simulink model "crazyflie"  (R2018b)
settings: Solver=VariableStepAuto  StartTime=0.0  StopTime=40  FixedStep=Ts  RelTol=1e-10
values from neighbouring files (symbols this model uses):
  bf = 1.28192e-08    [matlab.mat]    (also in model_init.m; work.mat)
  bm = 8.06428e-05    [matlab.mat]    (also in model_init.m; work.mat)
  c_10 = 0.5    [matlab.mat]    (also in model_init.m; work.mat)
  c_11 = 2    [matlab.mat]    (also in model_init.m; work.mat)
  c_12 = 0.5    [matlab.mat]    (also in model_init.m; work.mat)
  c_9 = 2    [matlab.mat]    (also in model_init.m; work.mat)
  g = 9.81    [matlab.mat]    (also in model_init.m; work.mat)
  Ix = 1.657171e-05    [matlab.mat]    (also in model_init.m; work.mat)
  Iy = 1.657171e-05    [matlab.mat]    (also in model_init.m; work.mat)
  Iz = 2.9261652e-05    [matlab.mat]    (also in model_init.m; work.mat)
  kdp = 0.03    [matlab.mat]    (also in model_init.m = 0.1; work.mat = 0.1)
  kdps = 0.01    [matlab.mat]    (also in model_init.m = 0.001; work.mat = 0.001)
  kdt = 0.03    [matlab.mat]    (also in model_init.m = 0.1; work.mat = 0.1)
  kdz = 3    [matlab.mat]    (also in model_init.m = 8; work.mat = 8)
  kiz = 2    [matlab.mat]    (also in model_init.m = 3; work.mat = 3)
  kpp = 0.03    [matlab.mat]    (also in model_init.m = 0.2; work.mat = 0.2)
  kpps = 0.01    [matlab.mat]    (also in model_init.m = 0.001; work.mat = 0.001)
  kpt = 0.03    [matlab.mat]    (also in model_init.m = 1; work.mat = 1)
  kpz = 2    [matlab.mat]    (also in model_init.m = 15; work.mat = 15)
  l = 0.046    [matlab.mat]    (also in model_init.m; work.mat)
  lambda_5 = 0.015    [matlab.mat]    (also in model_init.m; work.mat)
  lambda_6 = 0.015    [matlab.mat]    (also in model_init.m; work.mat)
  m = 0.027    [matlab.mat]    (also in model_init.m; work.mat)
  phi_ic = phi(end)    [Crazyflie_simulation.m]    (also in work.mat = 1.92698500832e-08)
  psi_ic = psi(end)    [Crazyflie_simulation.m]    (also in work.mat = 2.27785803884e-19)
  psi_r = 0    [Crazyflie_simulation.m]    (also in work.mat)
  sigma1_ic = sigma_1(end)    [Crazyflie_simulation.m]    (also in work.mat = 2272.7745434)
  sigma2_ic = sigma_2(end)    [Crazyflie_simulation.m]    (also in work.mat = 2272.7745434)
  sigma3_ic = sigma_3(end)    [Crazyflie_simulation.m]    (also in work.mat = 2272.77454331)
  sigma4_ic = sigma_4(end)    [Crazyflie_simulation.m]    (also in work.mat = 2272.77454331)
  Sigma_max = 2618    [matlab.mat]    (also in model_init.m; work.mat)
  T_m = 0.0125    [matlab.mat]    (also in model_init.m; work.mat)
  theta_ic = theta(end)    [Crazyflie_simulation.m]    (also in work.mat = 4.295907714e-08)
  x_ic = x(end)    [Crazyflie_simulation.m]    (also in work.mat = -0.000112604495344)
  x_r = 10*rrt_trajectory(i,1)/map_dimension(1)    [Crazyflie_simulation.m]    (also in matlab.mat = 1; work.mat = 0)
  y_ic = y(end)    [Crazyflie_simulation.m]    (also in work.mat = 9.00005076367)
  y_r = 10*rrt_trajectory(i,2)/map_dimension(2)    [Crazyflie_simulation.m]    (also in matlab.mat = 1; work.mat = 9)
  z_ic = z(end)    [Crazyflie_simulation.m]    (also in work.mat = 0.999916821767)
  z_r = 1    [Crazyflie_simulation.m]    (also in work.mat)
settings Model: Creator=alessandrosebastianelli  LastModifiedBy=alessandrosebastianelli
settings SFSimCC: SimUseLocalCustomCode=off
settings RTWCC: RTWUseLocalCustomCode=off

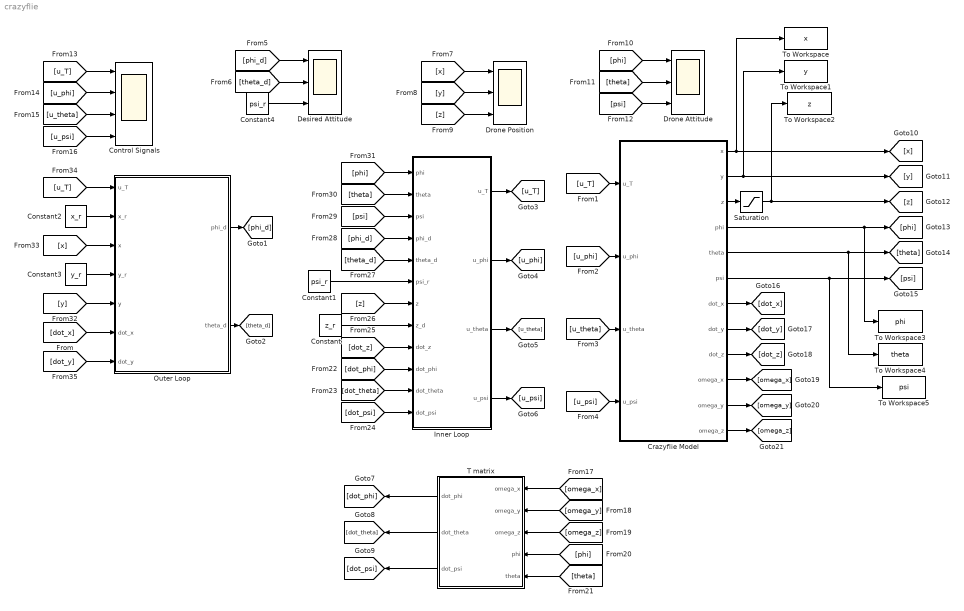
== system crazyflie ==
  Constant : Constant  Value=z_r
  Constant1 : Constant  Value=psi_r
  Constant2 : Constant  Value=x_r
  Constant3 : Constant  Value=y_r
  Constant4 : Constant  Value=psi_r
  Control Signals : Scope  NumInputPorts=4
  Crazyflie Model : Subsystem
  Desired Attitude : Scope  NumInputPorts=3
  Drone Attitude : Scope  NumInputPorts=3
  Drone Position : Scope  NumInputPorts=3
  Inner Loop : Subsystem
  Outer Loop : Subsystem
  Saturation : Saturate  UpperLimit=inf  LowerLimit=0
  T matrix : Subsystem
  To Workspace : ToWorkspace  VariableName=x  SampleTime=-1
  To Workspace1 : ToWorkspace  VariableName=y  SampleTime=-1
  To Workspace2 : ToWorkspace  VariableName=z  SampleTime=-1
  To Workspace3 : ToWorkspace  VariableName=phi  SampleTime=-1
  To Workspace4 : ToWorkspace  VariableName=theta  SampleTime=-1
  To Workspace5 : ToWorkspace  VariableName=psi  SampleTime=-1
  wires:
  Constant1/1 -> Inner Loop/6(psi_r)
  [dot_x] -> Outer Loop/6(dot_x)
  Outer Loop/2(theta_d) -> [theta_d]
  T matrix/1(dot_phi) -> [dot_phi]
  T matrix/2(dot_theta) -> [dot_theta]
  T matrix/3(dot_psi) -> [dot_psi]
  Inner Loop/1(u_T) -> [u_T]
  Inner Loop/2(u_phi) -> [u_phi]
  Inner Loop/3(u_theta) -> [u_theta]
  Inner Loop/4(u_psi) -> [u_psi]
  [u_T] -> Crazyflie Model/1(u_T)
  [u_phi] -> Crazyflie Model/2(u_phi)
  [u_theta] -> Crazyflie Model/3(u_theta)
  [u_psi] -> Crazyflie Model/4(u_psi)
  Crazyflie Model/1(x) -> [x], To Workspace/1
  Crazyflie Model/2(y) -> To Workspace1/1, [y]
  Crazyflie Model/3(z) -> Saturation/1
  Crazyflie Model/4(phi) -> To Workspace3/1, [phi]
  Crazyflie Model/5(theta) -> To Workspace4/1, [theta]
  Crazyflie Model/6(psi) -> To Workspace5/1, [psi]
  Crazyflie Model/7(dot_x) -> [dot_x]
  Crazyflie Model/8(dot_y) -> [dot_y]
  Crazyflie Model/9(dot_z) -> [dot_z]
  Crazyflie Model/10(omega_x) -> [omega_x]
  Crazyflie Model/11(omega_y) -> [omega_y]
  Crazyflie Model/12(omega_z) -> [omega_z]
  [phi_d] -> Desired Attitude/1
  [theta_d] -> Desired Attitude/2
  Constant4/1 -> Desired Attitude/3
  [z] -> Drone Position/3
  [y] -> Drone Position/2
  [x] -> Drone Position/1
  [phi] -> Drone Attitude/1
  [theta] -> Drone Attitude/2
  [psi] -> Drone Attitude/3
  [u_T] -> Control Signals/1
  [u_phi] -> Control Signals/2
  [u_theta] -> Control Signals/3
  [u_psi] -> Control Signals/4
  [omega_y] -> T matrix/2(omega_y)
  [omega_x] -> T matrix/1(omega_x)
  [omega_z] -> T matrix/3(omega_z)
  [phi] -> T matrix/4(phi)
  [theta] -> T matrix/5(theta)
  [dot_phi] -> Inner Loop/10(dot_phi)
  [dot_psi] -> Inner Loop/12(dot_psi)
  [dot_theta] -> Inner Loop/11(dot_theta)
  [dot_z] -> Inner Loop/9(dot_z)
  [z] -> Inner Loop/7(z)
  [phi] -> Inner Loop/1(phi)
  [theta] -> Inner Loop/2(theta)
  [psi] -> Inner Loop/3(psi)
  [phi_d] -> Inner Loop/4(phi_d)
  [theta_d] -> Inner Loop/5(theta_d)
  [u_T] -> Outer Loop/1("u_T ")
  [x] -> Outer Loop/3(x)
  [y] -> Outer Loop/5(y)
  Outer Loop/1(phi_d) -> [phi_d]
  [dot_y] -> Outer Loop/7(dot_y)
  Saturation/1 -> To Workspace2/1, [z]
  Constant2/1 -> Outer Loop/2(x_r)
  Constant3/1 -> Outer Loop/4(y_r)
  Constant/1 -> Inner Loop/8(z_d)

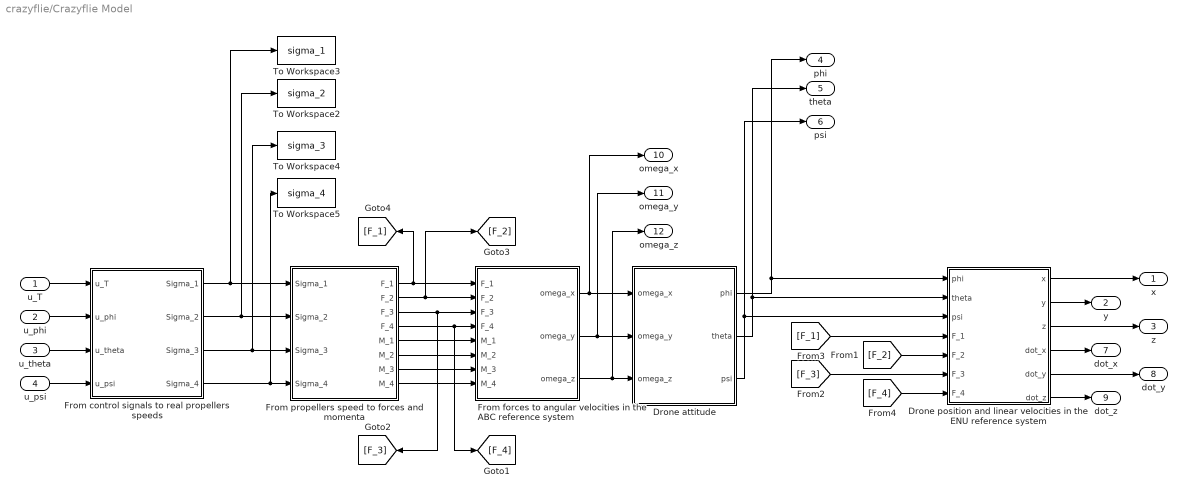
== system crazyflie/Crazyflie Model ==
  u_T : Inport
  u_phi : Inport  Port=2
  u_theta : Inport  Port=3
  u_psi : Inport  Port=4
  Drone attitude : Subsystem
  Drone position and linear velocities in the ENU reference system : Subsystem
  From control signals to real propellers speeds : Subsystem
  From forces to angular velocities in the ABC reference system : Subsystem
  From propellers speed to forces and momenta : Subsystem
  To Workspace2 : ToWorkspace  VariableName=sigma_2  SampleTime=-1
  To Workspace3 : ToWorkspace  VariableName=sigma_1  SampleTime=-1
  To Workspace4 : ToWorkspace  VariableName=sigma_3  SampleTime=-1
  To Workspace5 : ToWorkspace  VariableName=sigma_4  SampleTime=-1
  x : Outport
  y : Outport  Port=2
  z : Outport  Port=3
  phi : Outport  Port=4
  theta : Outport  Port=5
  psi : Outport  Port=6
  dot_x : Outport  Port=7
  dot_y : Outport  Port=8
  dot_z : Outport  Port=9
  omega_x : Outport  Port=10
  omega_y : Outport  Port=11
  omega_z : Outport  Port=12
  wires:
  u_T/1 -> From control signals to real propellers speeds/1(u_T)
  u_phi/1 -> From control signals to real propellers speeds/2(u_phi)
  u_theta/1 -> From control signals to real propellers speeds/3(u_theta)
  u_psi/1 -> From control signals to real propellers speeds/4(u_psi)
  From control signals to real propellers speeds/1(Sigma_1) -> To Workspace3/1, From propellers speed to forces and momenta/1(Sigma_1)
  From control signals to real propellers speeds/2(Sigma_2) -> To Workspace2/1, From propellers speed to forces and momenta/2(Sigma_2)
  From control signals to real propellers speeds/3(Sigma_3) -> To Workspace4/1, From propellers speed to forces and momenta/3(Sigma_3)
  From control signals to real propellers speeds/4(Sigma_4) -> To Workspace5/1, From propellers speed to forces and momenta/4(Sigma_4)
  From propellers speed to forces and momenta/1(F_1) -> [F_1], From forces to angular velocities in the ABC reference system/1(F_1)
  From propellers speed to forces and momenta/2(F_2) -> [F_2], From forces to angular velocities in the ABC reference system/2(F_2)
  From propellers speed to forces and momenta/3(F_3) -> [F_3], From forces to angular velocities in the ABC reference system/3(F_3)
  From propellers speed to forces and momenta/4(F_4) -> [F_4], From forces to angular velocities in the ABC reference system/4(F_4)
  From propellers speed to forces and momenta/5(M_1) -> From forces to angular velocities in the ABC reference system/5(M_1)
  From propellers speed to forces and momenta/6(M_2) -> From forces to angular velocities in the ABC reference system/6(M_2)
  From propellers speed to forces and momenta/7(M_3) -> From forces to angular velocities in the ABC reference system/7(M_3)
  From propellers speed to forces and momenta/8(M_4) -> From forces to angular velocities in the ABC reference system/8(M_4)
  From forces to angular velocities in the ABC reference system/1(omega_x) -> omega_x/1, Drone attitude/1(omega_x)
  From forces to angular velocities in the ABC reference system/2(omega_y) -> omega_y/1, Drone attitude/2(omega_y)
  From forces to angular velocities in the ABC reference system/3(omega_z) -> omega_z/1, Drone attitude/3(omega_z)
  Drone position and linear velocities in the ENU reference system/1(x) -> x/1
  Drone position and linear velocities in the ENU reference system/2(y) -> y/1
  Drone position and linear velocities in the ENU reference system/3(z) -> z/1
  Drone position and linear velocities in the ENU reference system/4(dot_x) -> dot_x/1
  Drone position and linear velocities in the ENU reference system/5(dot_y) -> dot_y/1
  Drone position and linear velocities in the ENU reference system/6(dot_z) -> dot_z/1
  Drone attitude/1(phi) -> Drone position and linear velocities in the ENU reference system/1(phi), phi/1
  Drone attitude/2(theta) -> Drone position and linear velocities in the ENU reference system/2(theta), theta/1
  Drone attitude/3(psi) -> Drone position and linear velocities in the ENU reference system/3(psi), psi/1
  [F_1] -> Drone position and linear velocities in the ENU reference system/4(F_1)
  [F_2] -> Drone position and linear velocities in the ENU reference system/5(F_2)
  [F_3] -> Drone position and linear velocities in the ENU reference system/6(F_3)
  [F_4] -> Drone position and linear velocities in the ENU reference system/7(F_4)

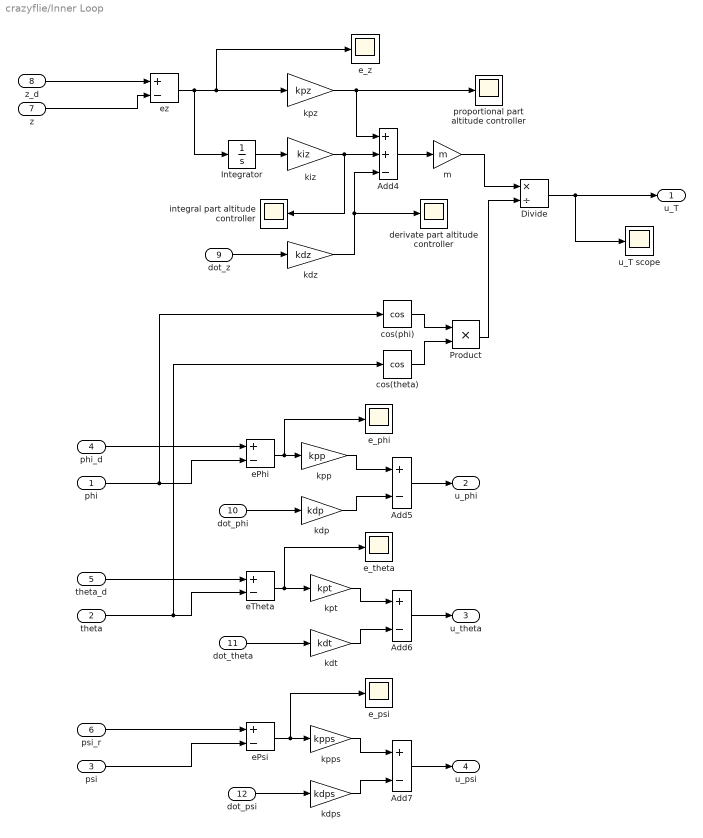
== system crazyflie/Inner Loop ==
  phi : Inport
  theta : Inport  Port=2
  psi : Inport  Port=3
  phi_d : Inport  Port=4
  theta_d : Inport  Port=5
  psi_r : Inport  Port=6
  z : Inport  Port=7
  z_d : Inport  Port=8
  dot_z : Inport  Port=9
  dot_phi : Inport  Port=10
  dot_theta : Inport  Port=11
  dot_psi : Inport  Port=12
  Add4 : Sum  Inputs=++-
  Add5 : Sum  Inputs=+-
  Add6 : Sum  Inputs=+-
  Add7 : Sum  Inputs=+-
  Divide : Product  Inputs=*/
  Integrator : Integrator
  Product : Product  RndMeth=Zero
  cos(phi) : Trigonometry  Operator=cos
  cos(theta) : Trigonometry  Operator=cos
  derivate part altitude controller : Scope
  ePhi : Sum  Inputs=+-
  ePsi : Sum  Inputs=+-
  eTheta : Sum  Inputs=+-
  e_phi : Scope
  e_psi : Scope
  e_theta : Scope
  e_z : Scope
  ez : Sum  Inputs=+-
  integral part altitude controller : Scope
  kdp : Gain  Gain=kdp
  kdps : Gain  Gain=kdps
  kdt : Gain  Gain=kdt
  kdz : Gain  Gain=kdz
  kiz : Gain  Gain=kiz
  kpp : Gain  Gain=kpp
  kpps : Gain  Gain=kpps
  kpt : Gain  Gain=kpt
  kpz : Gain  Gain=kpz
  m : Gain  Gain=m
  proportional part altitude controller : Scope
  u_T scope : Scope
  u_T : Outport
  u_phi : Outport  Port=2
  u_theta : Outport  Port=3
  u_psi : Outport  Port=4
  wires:
  phi/1 -> ePhi/2, cos(phi)/1
  theta/1 -> eTheta/2, cos(theta)/1
  psi/1 -> ePsi/2
  phi_d/1 -> ePhi/1
  theta_d/1 -> eTheta/1
  psi_r/1 -> ePsi/1
  ePhi/1 -> e_phi/1, kpp/1
  dot_phi/1 -> kdp/1
  eTheta/1 -> e_theta/1, kpt/1
  dot_theta/1 -> kdt/1
  ePsi/1 -> e_psi/1, kpps/1
  dot_psi/1 -> kdps/1
  z/1 -> ez/2
  z_d/1 -> ez/1
  ez/1 -> Integrator/1, kpz/1, e_z/1
  dot_z/1 -> kdz/1
  kpz/1 -> proportional part altitude controller/1, Add4/1
  kdz/1 -> Add4/3, derivate part altitude controller/1
  kpp/1 -> Add5/1
  kdp/1 -> Add5/2
  Add5/1 -> u_phi/1
  kpt/1 -> Add6/1
  kdt/1 -> Add6/2
  Add6/1 -> u_theta/1
  kpps/1 -> Add7/1
  kdps/1 -> Add7/2
  Add7/1 -> u_psi/1
  cos(phi)/1 -> Product/1
  cos(theta)/1 -> Product/2
  Add4/1 -> m/1
  m/1 -> Divide/1
  Product/1 -> Divide/2
  Divide/1 -> u_T/1, u_T scope/1
  kiz/1 -> integral part altitude controller/1, Add4/2
  Integrator/1 -> kiz/1

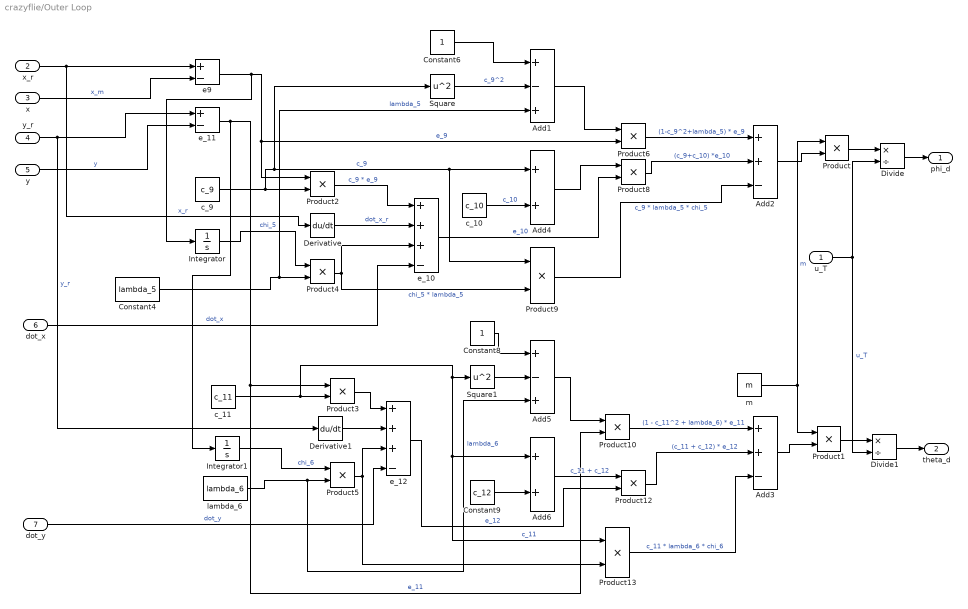
== system crazyflie/Outer Loop ==
  "u_T " : Inport
  x_r : Inport  Port=2
  x : Inport  Port=3
  y_r : Inport  Port=4
  y : Inport  Port=5
  dot_x : Inport  Port=6
  dot_y : Inport  Port=7
  Add1 : Sum  Inputs=+-+
  Add2 : Sum  Inputs=++-
  Add3 : Sum  Inputs=++-
  Add4 : Sum
  Add5 : Sum  Inputs=+-+
  Add6 : Sum
  Constant4 : Constant  Value=lambda_5
  Constant6 : Constant
  Constant8 : Constant
  Constant9 : Constant  Value=c_12
  Derivative : Derivative
  Derivative1 : Derivative
  Divide : Product  Inputs=*/
  Divide1 : Product  Inputs=*/
  Integrator : Integrator
  Integrator1 : Integrator
  Product{,1..6,8..10,12..13} (12 alike) : Product
  Square : Math  Operator=square  SaturateOnIntegerOverflow=on
  Square1 : Math  Operator=square  SaturateOnIntegerOverflow=on
  c_10 : Constant  Value=c_10
  c_11 : Constant  Value=c_11
  c_9 : Constant  Value=c_9
  e9 : Sum  Inputs=+-
  e_10 : Sum  Inputs=+++-
  e_11 : Sum  Inputs=+-
  e_12 : Sum  Inputs=+++-
  lambda_6 : Constant  Value=lambda_6
  m : Constant  Value=m
  phi_d : Outport
  theta_d : Outport  Port=2
  wires:
  x_r/1 -> Derivative/1, e9/1  "x_r"
  x/1 -> e9/2  "x_m"
  y_r/1 -> Derivative1/1, e_11/1  "y_r"
  y/1 -> e_11/2  "y"
  Product/1 -> Divide/1
  m/1 -> Product/1, Product1/1  "m"
  "u_T "/1 -> Divide/2, Divide1/2  "u_T"
  Product1/1 -> Divide1/1
  Divide/1 -> phi_d/1
  Divide1/1 -> theta_d/1
  Add2/1 -> Product/2
  Add3/1 -> Product1/2
  Product2/1 -> e_10/1  "c_9 * e_9"
  c_9/1 -> Product2/2, Square/1, Product9/1, Add4/1  "c_9"
  e9/1 -> Integrator/1, Product2/1, Product6/2  "e_9"
  Product3/1 -> e_12/1
  c_11/1 -> Product3/2, Square1/1, Product13/1, Add6/1  "c_11"
  e_11/1 -> Product10/2, Product3/1, Integrator1/1  "e_11"
  Product4/1 -> Product9/2, e_10/3  "chi_5 * lambda_5"
  Constant4/1 -> Add1/3, Product4/2  "lambda_5"
  Product5/1 -> e_12/3, Product13/2
  lambda_6/1 -> Product5/2, Add5/3  "lambda_6"
  Product6/1 -> Add2/1  "(1-c_9^2+lambda_5) * e_9"
  Add1/1 -> Product6/1
  Constant6/1 -> Add1/1
  Square/1 -> Add1/2  "c_9^2"
  Product8/1 -> Add2/2  "(c_9+c_10) *e_10"
  e_10/1 -> Product8/2  "e_10"
  Add4/1 -> Product8/1
  c_10/1 -> Add4/2  "c_10"
  Product9/1 -> Add2/3  "c_9 * lambda_5 * chi_5"
  Add5/1 -> Product10/1
  Square1/1 -> Add5/2
  Constant8/1 -> Add5/1
  Product10/1 -> Add3/1  "(1 - c_11^2 + lambda_6) * e_11"
  Constant9/1 -> Add6/2
  Product12/1 -> Add3/2  "(c_11 + c_12) * e_12"
  Add6/1 -> Product12/1  "c_11 + c_12"
  e_12/1 -> Product12/2  "e_12"
  Product13/1 -> Add3/3  "c_11 * lambda_6 * chi_6"
  Integrator/1 -> Product4/1  "chi_5"
  Integrator1/1 -> Product5/1  "chi_6"
  Derivative/1 -> e_10/2  "dot_x_r"
  dot_x/1 -> e_10/4  "dot_x"
  Derivative1/1 -> e_12/2
  dot_y/1 -> e_12/4  "dot_y"

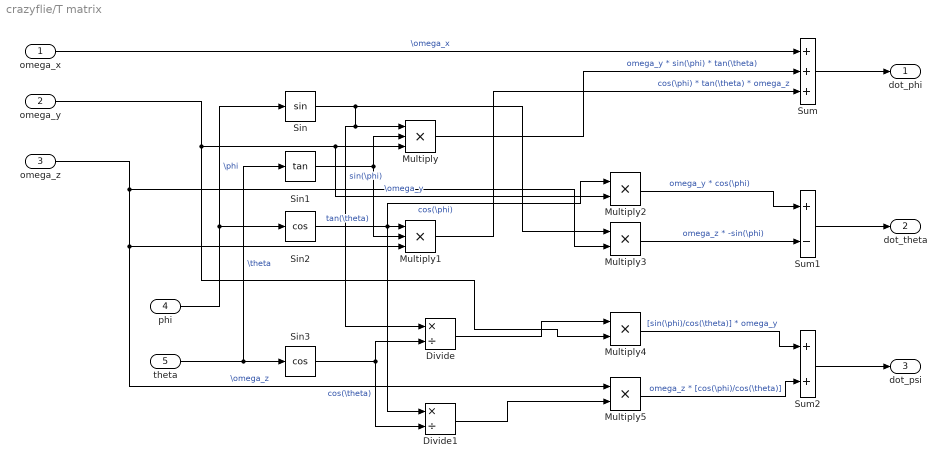
== system crazyflie/T matrix ==
  omega_x : Inport
  omega_y : Inport  Port=2
  omega_z : Inport  Port=3
  phi : Inport  Port=4
  theta : Inport  Port=5
  Divide : Product  Inputs=*/
  Divide1 : Product  Inputs=*/
  Multiply : Product  Inputs=3
  Multiply1 : Product  Inputs=3
  Multiply{2..5} (4 alike) : Product
  Sin : Trigonometry
  Sin1 : Trigonometry  Operator=tan
  Sin2 : Trigonometry  Operator=cos
  Sin3 : Trigonometry  Operator=cos
  Sum : Sum  Inputs=+++
  Sum1 : Sum  Inputs=+-
  Sum2 : Sum
  dot_phi : Outport
  dot_theta : Outport  Port=2
  dot_psi : Outport  Port=3
  wires:
  Sum/1 -> dot_phi/1
  Sum1/1 -> dot_theta/1
  Sum2/1 -> dot_psi/1
  omega_x/1 -> Sum/1  "\\omega_x"
  Sin/1 -> Multiply3/1, Divide/1, Multiply/1  "sin(\\phi)"
  Sin1/1 -> Multiply1/2, Multiply/2  "tan(\\theta)"
  phi/1 -> Sin2/1, Sin/1  "\\phi"
  theta/1 -> Sin3/1, Sin1/1  "\\theta"
  omega_y/1 -> Multiply2/2, Multiply/3, Multiply4/2  "\\omega_y"
  Multiply/1 -> Sum/2  "omega_y * sin(\\phi) * tan(\\theta)"
  Sin2/1 -> Multiply2/1, Divide1/1, Multiply1/1  "cos(\\phi)"
  Multiply1/1 -> Sum/3  "cos(\\phi) * tan(\\theta) * omega_z"
  Multiply2/1 -> Sum1/1  "omega_y * cos(\\phi)"
  Multiply3/1 -> Sum1/2  "omega_z * -sin(\\phi)"
  omega_z/1 -> Multiply3/2, Multiply1/3, Multiply5/1  "\\omega_z"
  Multiply4/1 -> Sum2/1  "[sin(\\phi)/cos(\\theta)] * omega_y"
  Multiply5/1 -> Sum2/2  "omega_z * [cos(\\phi)/cos(\\theta)]"
  Sin3/1 -> Divide1/2, Divide/2  "cos(\\theta)"
  Divide/1 -> Multiply4/1
  Divide1/1 -> Multiply5/2

== system crazyflie/Crazyflie Model/Drone attitude ==
  omega_x : Inport
  omega_y : Inport  Port=2
  omega_z : Inport  Port=3
  T matrix : Subsystem
  phi integrator : Integrator  InitialCondition=phi_ic
  psi integrator : Integrator  InitialCondition=psi_ic
  theta integrator : Integrator  InitialCondition=theta_ic
  phi : Outport
  theta : Outport  Port=2
  psi : Outport  Port=3
  wires:
  phi integrator/1 -> [phi], phi/1
  theta integrator/1 -> theta/1, [theta]
  psi integrator/1 -> psi/1
  omega_x/1 -> T matrix/1(omega_x)
  omega_y/1 -> T matrix/2(omega_y)
  omega_z/1 -> T matrix/3(omega_z)
  [theta] -> T matrix/5(theta)
  [phi] -> T matrix/4(phi)
  T matrix/1(dot_phi) -> phi integrator/1
  T matrix/2(dot_theta) -> theta integrator/1
  T matrix/3(dot_psi) -> psi integrator/1

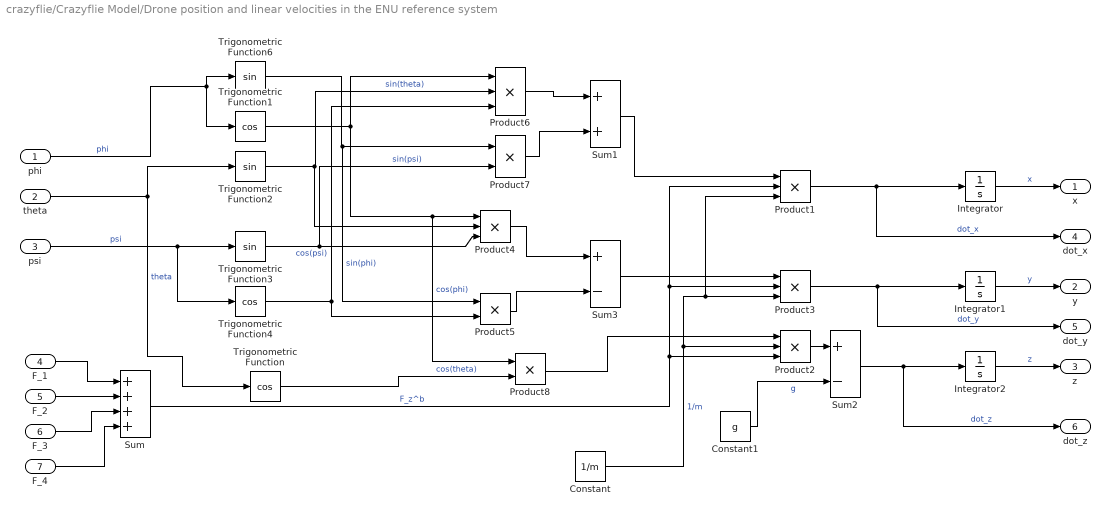
== system crazyflie/Crazyflie Model/Drone position and linear velocities in the ENU reference system ==
  phi : Inport
  theta : Inport  Port=2
  psi : Inport  Port=3
  F_1 : Inport  Port=4
  F_2 : Inport  Port=5
  F_3 : Inport  Port=6
  F_4 : Inport  Port=7
  Constant : Constant  Value=1/m
  Constant1 : Constant  Value=g
  Integrator : Integrator  InitialCondition=x_ic
  Integrator1 : Integrator  InitialCondition=y_ic
  Integrator2 : Integrator  InitialCondition=z_ic
  Product{1..4,6} (5 alike) : Product  Inputs=3
  Product5 : Product
  Product7 : Product
  Product8 : Product
  Sum : Sum  Inputs=++++
  Sum1 : Sum
  Sum2 : Sum  Inputs=+-
  Sum3 : Sum  Inputs=+-
  Trigonometric Function : Trigonometry  Operator=cos
  Trigonometric Function1 : Trigonometry  Operator=cos
  Trigonometric Function2 : Trigonometry
  Trigonometric Function3 : Trigonometry
  Trigonometric Function4 : Trigonometry  Operator=cos
  Trigonometric Function6 : Trigonometry
  x : Outport
  y : Outport  Port=2
  z : Outport  Port=3
  dot_x : Outport  Port=4
  dot_y : Outport  Port=5
  dot_z : Outport  Port=6
  wires:
  F_1/1 -> Sum/1
  F_2/1 -> Sum/2
  F_3/1 -> Sum/3
  F_4/1 -> Sum/4
  Integrator/1 -> x/1  "x"
  Integrator1/1 -> y/1  "y"
  Integrator2/1 -> z/1  "z"
  theta/1 -> Trigonometric Function2/1, Trigonometric Function/1  "theta"
  Constant/1 -> Product1/3, Product3/3, Product2/2  "1/m"
  Product2/1 -> Sum2/1
  Constant1/1 -> Sum2/2  "g"
  Sum/1 -> Product1/2, Product3/2, Product2/3  "F_z^b"
  Sum2/1 -> dot_z/1, Integrator2/1  "dot_z"
  Sum3/1 -> Product3/1
  Product4/1 -> Sum3/1
  Product3/1 -> Integrator1/1, dot_y/1  "dot_y"
  Product5/1 -> Sum3/2
  Product1/1 -> dot_x/1, Integrator/1  "dot_x"
  Sum1/1 -> Product1/1
  Product6/1 -> Sum1/1
  Product7/1 -> Sum1/2
  phi/1 -> Trigonometric Function1/1, Trigonometric Function6/1  "phi"
  psi/1 -> Trigonometric Function3/1, Trigonometric Function4/1  "psi"
  Trigonometric Function1/1 -> Product8/1, Product4/1, Product6/1  "cos(phi)"
  Trigonometric Function2/1 -> Product4/2, Product6/2  "sin(theta)"
  Trigonometric Function4/1 -> Product5/2, Product6/3  "cos(psi)"
  Trigonometric Function6/1 -> Product5/1, Product7/1  "sin(phi)"
  Trigonometric Function3/1 -> Product7/2, Product4/3  "sin(psi)"
  Trigonometric Function/1 -> Product8/2  "cos(theta)"
  Product8/1 -> Product2/1

== system crazyflie/Crazyflie Model/From control signals to real propellers speeds ==
  u_T : Inport
  u_phi : Inport  Port=2
  u_theta : Inport  Port=3
  u_psi : Inport  Port=4
  Dai segnali di controllo alle velocità angolari dei rotori : Subsystem  Commented=on
  Desired Omega Values : Scope  NumInputPorts=4
  From control signals to propellers angular velocities : Subsystem
  Motors dynamics : Subsystem
  Scope1 : Scope  NumInputPorts=4
  Sigma_1 : Outport
  Sigma_2 : Outport  Port=2
  Sigma_3 : Outport  Port=3
  Sigma_4 : Outport  Port=4
  wires:
  u_T/1 -> From control signals to propellers angular velocities/1(u_T)
  From control signals to propellers angular velocities/1(Sigma_1_d) -> Motors dynamics/1(Sigma_1_d), Desired Omega Values/1
  From control signals to propellers angular velocities/2(Sigma_2_d) -> Desired Omega Values/2, Motors dynamics/2(Sigma_2_d)
  From control signals to propellers angular velocities/3(Sigma_3_d) -> Desired Omega Values/3, Motors dynamics/3(Sigma_3_d)
  From control signals to propellers angular velocities/4(Sigma_4_d) -> Desired Omega Values/4, Motors dynamics/4(Sigma_4_d)
  u_phi/1 -> From control signals to propellers angular velocities/2(u_phi)
  u_theta/1 -> From control signals to propellers angular velocities/3(u_theta)
  u_psi/1 -> From control signals to propellers angular velocities/4(u_psi)
  Motors dynamics/4(Sigma_4) -> Scope1/4, Sigma_4/1
  Motors dynamics/3(Sigma_3) -> Scope1/3, Sigma_3/1
  Motors dynamics/2(Sigma_2) -> Scope1/2, Sigma_2/1
  Motors dynamics/1(Sigma_1) -> Scope1/1, Sigma_1/1

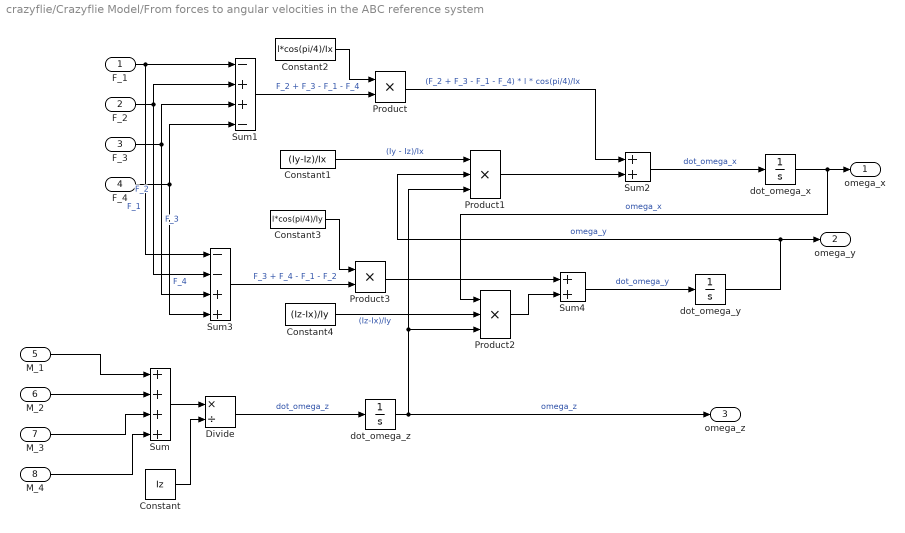
== system crazyflie/Crazyflie Model/From forces to angular velocities in the ABC reference system ==
  F_1 : Inport
  F_2 : Inport  Port=2
  F_3 : Inport  Port=3
  F_4 : Inport  Port=4
  M_1 : Inport  Port=5
  M_2 : Inport  Port=6
  M_3 : Inport  Port=7
  M_4 : Inport  Port=8
  Constant : Constant  Value=Iz
  Constant1 : Constant  Value=(Iy-Iz)/Ix
  Constant2 : Constant  Value=l*cos(pi/4)/Ix
  Constant3 : Constant  Value=l*cos(pi/4)/Iy
  Constant4 : Constant  Value=(Iz-Ix)/Iy
  Divide : Product  Inputs=*/
  Product : Product
  Product1 : Product  Inputs=3
  Product2 : Product  Inputs=3
  Product3 : Product
  Sum : Sum  Inputs=++++
  Sum1 : Sum  Inputs=-++-
  Sum2 : Sum
  Sum3 : Sum  Inputs=--++
  Sum4 : Sum
  dot_omega_x : Integrator
  dot_omega_y : Integrator
  dot_omega_z : Integrator
  omega_x : Outport
  omega_y : Outport  Port=2
  omega_z : Outport  Port=3
  wires:
  M_1/1 -> Sum/1
  M_2/1 -> Sum/2
  M_3/1 -> Sum/3
  M_4/1 -> Sum/4
  Sum/1 -> Divide/1
  Constant/1 -> Divide/2
  Divide/1 -> dot_omega_z/1  "dot_omega_z"
  F_1/1 -> Sum1/1, Sum3/1  "F_1"
  F_2/1 -> Sum3/2, Sum1/2  "F_2"
  F_3/1 -> Sum3/3, Sum1/3  "F_3"
  F_4/1 -> Sum3/4, Sum1/4  "F_4"
  Constant1/1 -> Product1/1  "(Iy - Iz)/Ix"
  dot_omega_z/1 -> omega_z/1, Product1/3, Product2/3  "omega_z"
  Product1/1 -> Sum2/2
  Sum1/1 -> Product/2  "F_2 + F_3 - F_1 - F_4"
  Constant2/1 -> Product/1
  Product/1 -> Sum2/1  "(F_2 + F_3 - F_1 - F_4) * l * cos(pi/4)/Ix"
  Sum2/1 -> dot_omega_x/1  "dot_omega_x"
  Sum3/1 -> Product3/2  "F_3 + F_4 - F_1 - F_2"
  Constant3/1 -> Product3/1
  Product3/1 -> Sum4/1
  dot_omega_x/1 -> omega_x/1, Product2/1  "omega_x"
  Product2/1 -> Sum4/2
  Sum4/1 -> dot_omega_y/1  "dot_omega_y"
  dot_omega_y/1 -> Product1/2, omega_y/1  "omega_y"
  Constant4/1 -> Product2/2  "(Iz-Ix)/Iy"

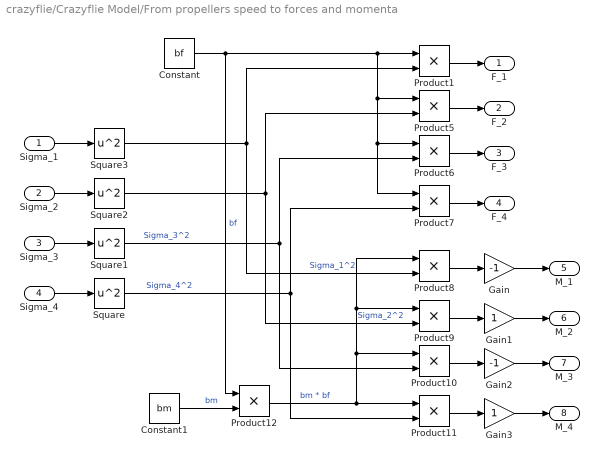
== system crazyflie/Crazyflie Model/From propellers speed to forces and momenta ==
  Sigma_1 : Inport
  Sigma_2 : Inport  Port=2
  Sigma_3 : Inport  Port=3
  Sigma_4 : Inport  Port=4
  Constant : Constant  Value=bf
  Constant1 : Constant  Value=bm
  Gain : Gain  Gain=-1
  Gain1 : Gain
  Gain2 : Gain  Gain=-1
  Gain3 : Gain
  Product{1,5..12} (9 alike) : Product
  Square{,1..3} (4 alike) : Math  Operator=square  SaturateOnIntegerOverflow=on
  F_1 : Outport
  F_2 : Outport  Port=2
  F_3 : Outport  Port=3
  F_4 : Outport  Port=4
  M_1 : Outport  Port=5
  M_2 : Outport  Port=6
  M_3 : Outport  Port=7
  M_4 : Outport  Port=8
  wires:
  Sigma_1/1 -> Square3/1
  Sigma_2/1 -> Square2/1
  Sigma_3/1 -> Square1/1
  Sigma_4/1 -> Square/1
  Constant/1 -> Product5/1, Product6/1, Product7/1, Product1/1, Product12/1  "bf"
  Constant1/1 -> Product12/2  "bm"
  Product12/1 -> Product11/1, Product10/1, Product9/1, Product8/1  "bm * bf"
  Product1/1 -> F_1/1
  Product5/1 -> F_2/1
  Product6/1 -> F_3/1
  Product7/1 -> F_4/1
  Product9/1 -> Gain1/1
  Product11/1 -> Gain3/1
  Product8/1 -> Gain/1
  Product10/1 -> Gain2/1
  Square2/1 -> Product5/2, Product9/2  "Sigma_2^2"
  Square1/1 -> Product10/2, Product6/2  "Sigma_3^2"
  Square/1 -> Product7/2, Product11/2  "Sigma_4^2"
  Square3/1 -> Product8/2, Product1/2  "Sigma_1^2"
  Gain/1 -> M_1/1
  Gain1/1 -> M_2/1
  Gain2/1 -> M_3/1
  Gain3/1 -> M_4/1

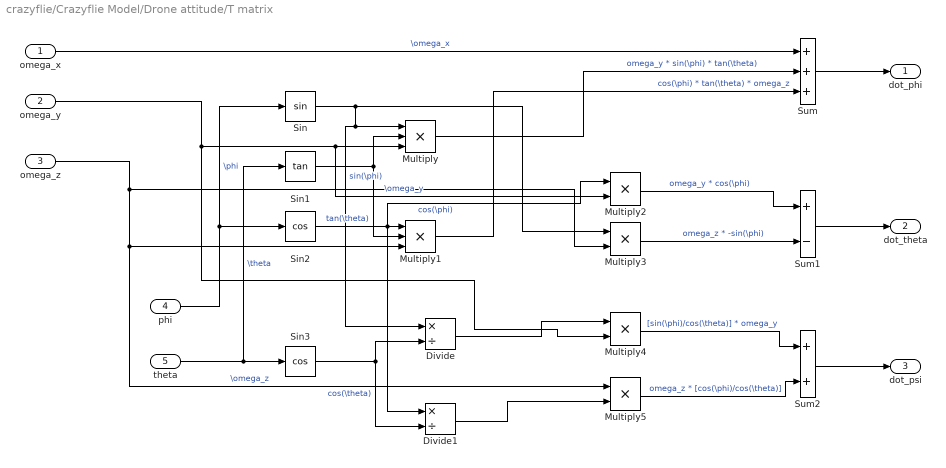
== system crazyflie/Crazyflie Model/Drone attitude/T matrix ==
  omega_x : Inport
  omega_y : Inport  Port=2
  omega_z : Inport  Port=3
  phi : Inport  Port=4
  theta : Inport  Port=5
  Divide : Product  Inputs=*/
  Divide1 : Product  Inputs=*/
  Multiply : Product  Inputs=3
  Multiply1 : Product  Inputs=3
  Multiply{2..5} (4 alike) : Product
  Sin : Trigonometry
  Sin1 : Trigonometry  Operator=tan
  Sin2 : Trigonometry  Operator=cos
  Sin3 : Trigonometry  Operator=cos
  Sum : Sum  Inputs=+++
  Sum1 : Sum  Inputs=+-
  Sum2 : Sum
  dot_phi : Outport
  dot_theta : Outport  Port=2
  dot_psi : Outport  Port=3
  wires:
  Sum/1 -> dot_phi/1
  Sum1/1 -> dot_theta/1
  Sum2/1 -> dot_psi/1
  omega_x/1 -> Sum/1  "\\omega_x"
  Sin/1 -> Multiply3/1, Divide/1, Multiply/1  "sin(\\phi)"
  Sin1/1 -> Multiply1/2, Multiply/2  "tan(\\theta)"
  phi/1 -> Sin2/1, Sin/1  "\\phi"
  theta/1 -> Sin3/1, Sin1/1  "\\theta"
  omega_y/1 -> Multiply2/2, Multiply/3, Multiply4/2  "\\omega_y"
  Multiply/1 -> Sum/2  "omega_y * sin(\\phi) * tan(\\theta)"
  Sin2/1 -> Multiply2/1, Divide1/1, Multiply1/1  "cos(\\phi)"
  Multiply1/1 -> Sum/3  "cos(\\phi) * tan(\\theta) * omega_z"
  Multiply2/1 -> Sum1/1  "omega_y * cos(\\phi)"
  Multiply3/1 -> Sum1/2  "omega_z * -sin(\\phi)"
  omega_z/1 -> Multiply3/2, Multiply1/3, Multiply5/1  "\\omega_z"
  Multiply4/1 -> Sum2/1  "[sin(\\phi)/cos(\\theta)] * omega_y"
  Multiply5/1 -> Sum2/2  "omega_z * [cos(\\phi)/cos(\\theta)]"
  Sin3/1 -> Divide1/2, Divide/2  "cos(\\theta)"
  Divide/1 -> Multiply4/1
  Divide1/1 -> Multiply5/2

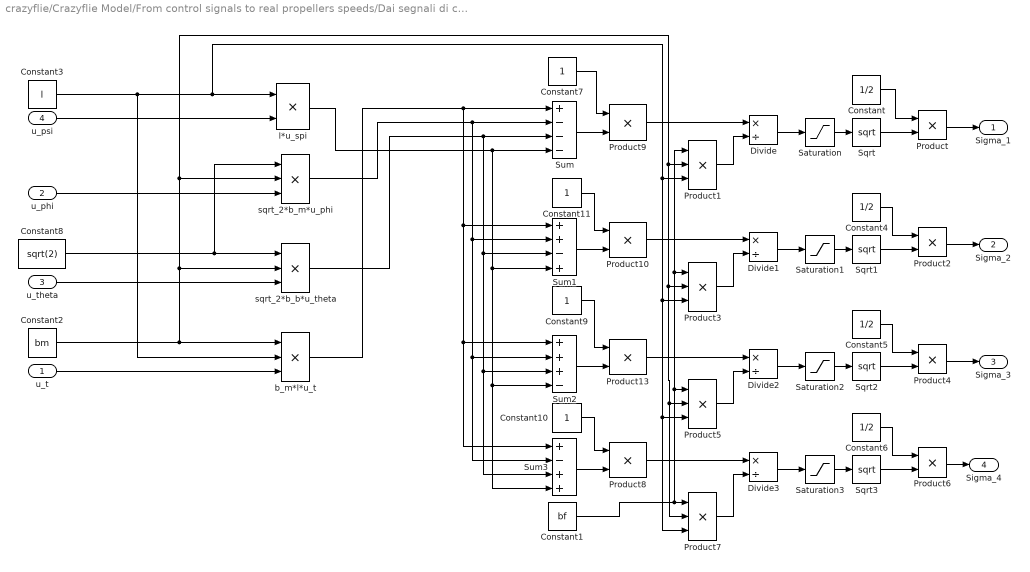
== system crazyflie/Crazyflie Model/From control signals to real propellers speeds/Dai segnali di controllo alle velocità angolari dei rotori ==
  u_t : Inport
  u_phi : Inport  Port=2
  u_theta : Inport  Port=3
  u_psi : Inport  Port=4
  Constant{,4..6} (4 alike) : Constant  Value=1/2
  Constant1 : Constant  Value=bf
  Constant{7,9..11} (4 alike) : Constant
  Constant2 : Constant  Value=bm
  Constant3 : Constant  Value=l
  Constant8 : Constant  Value=sqrt(2)
  Divide{,1..3} (4 alike) : Product  Inputs=*/
  Product{,2,4,6,8..10,13} (8 alike) : Product
  Product{1,3,5,7} (4 alike) : Product  Inputs=3
  Saturation{,1..3} (4 alike) : Saturate  UpperLimit=inf  LowerLimit=0
  Sqrt{,1..3} (4 alike) : Sqrt  SaturateOnIntegerOverflow=on
  Sum : Sum  Inputs=+---
  Sum1 : Sum  Inputs=++-+
  Sum2 : Sum  Inputs=+++-
  Sum3 : Sum  Inputs=+-++
  b_m*l*u_t : Product  Inputs=3
  l*u_spi : Product
  sqrt_2*b_b*u_theta : Product  Inputs=3
  sqrt_2*b_m*u_phi : Product  Inputs=3
  Sigma_1 : Outport
  Sigma_2 : Outport  Port=2
  Sigma_3 : Outport  Port=3
  Sigma_4 : Outport  Port=4
  wires:
  Constant/1 -> Product/1
  Product/1 -> Sigma_1/1
  Sqrt/1 -> Product/2
  Product1/1 -> Divide/2
  Constant2/1 -> Product7/2, Product5/2, Product3/2, Product1/2, sqrt_2*b_m*u_phi/2, sqrt_2*b_b*u_theta/2, b_m*l*u_t/1
  Constant3/1 -> b_m*l*u_t/2, Product7/3, Product5/3, Product3/3, Product1/3, l*u_spi/1
  Constant4/1 -> Product2/1
  Product3/1 -> Divide1/2
  Sqrt1/1 -> Product2/2
  Product2/1 -> Sigma_2/1
  Sqrt2/1 -> Product4/2
  Product5/1 -> Divide2/2
  Constant5/1 -> Product4/1
  Product4/1 -> Sigma_3/1
  Constant6/1 -> Product6/1
  Sqrt3/1 -> Product6/2
  Product7/1 -> Divide3/2
  Product6/1 -> Sigma_4/1
  Sum/1 -> Product9/2
  Product9/1 -> Divide/1
  Constant7/1 -> Product9/1
  Constant8/1 -> sqrt_2*b_m*u_phi/1, sqrt_2*b_b*u_theta/1
  u_psi/1 -> l*u_spi/2
  u_phi/1 -> sqrt_2*b_m*u_phi/3
  u_theta/1 -> sqrt_2*b_b*u_theta/3
  u_t/1 -> b_m*l*u_t/3
  Sum2/1 -> Product13/2
  Product13/1 -> Divide2/1
  Constant9/1 -> Product13/1
  Constant1/1 -> Product1/1, Product3/1, Product5/1, Product7/1
  Product8/1 -> Divide3/1
  Sum3/1 -> Product8/2
  Constant10/1 -> Product8/1
  Sum1/1 -> Product10/2
  Product10/1 -> Divide1/1
  Constant11/1 -> Product10/1
  Saturation/1 -> Sqrt/1
  Divide/1 -> Saturation/1
  Divide1/1 -> Saturation1/1
  Saturation1/1 -> Sqrt1/1
  Saturation2/1 -> Sqrt2/1
  Divide2/1 -> Saturation2/1
  Divide3/1 -> Saturation3/1
  Saturation3/1 -> Sqrt3/1
  b_m*l*u_t/1 -> Sum3/1, Sum2/1, Sum1/1, Sum/1
  sqrt_2*b_m*u_phi/1 -> Sum3/2, Sum2/2, Sum1/2, Sum/2
  sqrt_2*b_b*u_theta/1 -> Sum3/3, Sum2/3, Sum1/3, Sum/3
  l*u_spi/1 -> Sum3/4, Sum2/4, Sum1/4, Sum/4

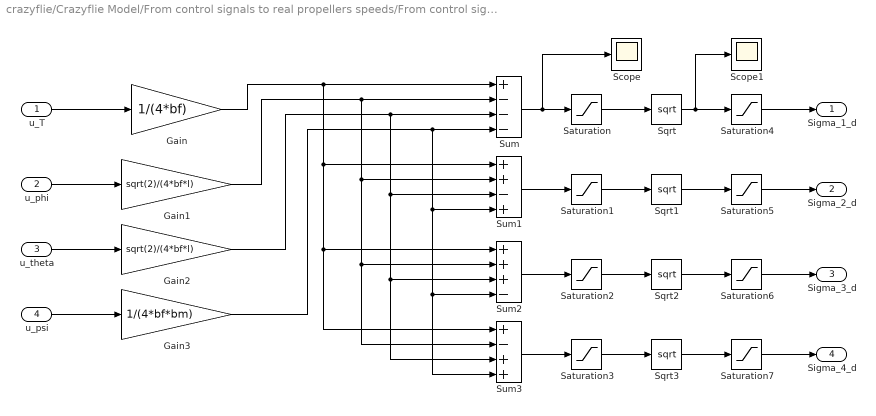
== system crazyflie/Crazyflie Model/From control signals to real propellers speeds/From control signals to propellers angular velocities ==
  u_T : Inport
  u_phi : Inport  Port=2
  u_theta : Inport  Port=3
  u_psi : Inport  Port=4
  Gain : Gain  Gain=1/(4*bf)
  Gain1 : Gain  Gain=sqrt(2)/(4*bf*l)
  Gain2 : Gain  Gain=sqrt(2)/(4*bf*l)
  Gain3 : Gain  Gain=1/(4*bf*bm)
  Saturation{,1..3} (4 alike) : Saturate  UpperLimit=inf  LowerLimit=0
  Saturation{4..7} (4 alike) : Saturate  UpperLimit=Sigma_max  LowerLimit=0
  Scope : Scope
  Scope1 : Scope
  Sqrt{,1..3} (4 alike) : Sqrt  SaturateOnIntegerOverflow=on
  Sum : Sum  Inputs=+---
  Sum1 : Sum  Inputs=++-+
  Sum2 : Sum  Inputs=+++-
  Sum3 : Sum  Inputs=+-++
  Sigma_1_d : Outport
  Sigma_2_d : Outport  Port=2
  Sigma_3_d : Outport  Port=3
  Sigma_4_d : Outport  Port=4
  wires:
  Sqrt1/1 -> Saturation5/1
  Sqrt2/1 -> Saturation6/1
  Sqrt3/1 -> Saturation7/1
  Saturation/1 -> Sqrt/1
  Saturation1/1 -> Sqrt1/1
  Sum1/1 -> Saturation1/1
  Sum/1 -> Scope/1, Saturation/1
  Saturation2/1 -> Sqrt2/1
  Sum2/1 -> Saturation2/1
  Saturation3/1 -> Sqrt3/1
  Sum3/1 -> Saturation3/1
  Sqrt/1 -> Scope1/1, Saturation4/1
  u_T/1 -> Gain/1
  u_phi/1 -> Gain1/1
  u_theta/1 -> Gain2/1
  u_psi/1 -> Gain3/1
  Gain/1 -> Sum/1, Sum1/1, Sum2/1, Sum3/1
  Gain1/1 -> Sum/2, Sum1/2, Sum2/2, Sum3/2
  Gain2/1 -> Sum/3, Sum1/3, Sum2/3, Sum3/3
  Gain3/1 -> Sum/4, Sum1/4, Sum2/4, Sum3/4
  Saturation4/1 -> Sigma_1_d/1
  Saturation5/1 -> Sigma_2_d/1
  Saturation6/1 -> Sigma_3_d/1
  Saturation7/1 -> Sigma_4_d/1

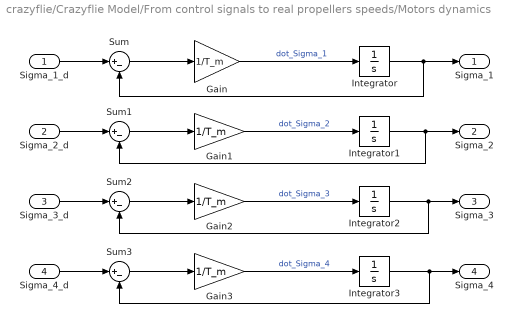
== system crazyflie/Crazyflie Model/From control signals to real propellers speeds/Motors dynamics ==
  Sigma_1_d : Inport
  Sigma_2_d : Inport  Port=2
  Sigma_3_d : Inport  Port=3
  Sigma_4_d : Inport  Port=4
  Gain{,1..3} (4 alike) : Gain  Gain=1/T_m
  Integrator : Integrator  InitialCondition=sigma1_ic
  Integrator1 : Integrator  InitialCondition=sigma2_ic
  Integrator2 : Integrator  InitialCondition=sigma3_ic
  Integrator3 : Integrator  InitialCondition=sigma4_ic
  Sum{,1..3} (4 alike) : Sum  Inputs=|+-
  Sigma_1 : Outport
  Sigma_2 : Outport  Port=2
  Sigma_3 : Outport  Port=3
  Sigma_4 : Outport  Port=4
  wires:
  Sigma_1_d/1 -> Sum/1
  Integrator3/1 -> Sum3/2, Sigma_4/1
  Sum3/1 -> Gain3/1
  Sum/1 -> Gain/1
  Integrator1/1 -> Sum1/2, Sigma_2/1
  Integrator/1 -> Sum/2, Sigma_1/1
  Sum1/1 -> Gain1/1
  Gain2/1 -> Integrator2/1  "dot_Sigma_3"
  Gain/1 -> Integrator/1  "dot_Sigma_1"
  Gain1/1 -> Integrator1/1  "dot_Sigma_2"
  Gain3/1 -> Integrator3/1  "dot_Sigma_4"
  Sum2/1 -> Gain2/1
  Integrator2/1 -> Sum2/2, Sigma_3/1
  Sigma_4_d/1 -> Sum3/1
  Sigma_2_d/1 -> Sum1/1
  Sigma_3_d/1 -> Sum2/1
